simulink model "int2single"  (Simulink 7.6)
settings: Solver=FixedStepDiscrete  StartTime=0.0  StopTime=10000  FixedStep=1  RelTol=1e-3
settings Model: Creator=jordan  LastModifiedBy=jordan
settings DataIOCC: LimitDataPoints=off  SaveOutput=off  SignalLogging=off  DSMLogging=off  SaveTime=off
settings OptimizationCC: BlockReduction=off  ConditionallyExecuteInputs=off

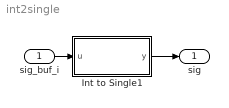
== system int2single ==
  sig_buf_i : Inport  OutDataTypeStr=fixdt(0,12,0)
  Int to Single1 : Stateflow chart  TreatAsAtomicUnit=on
  sig : Outport  OutDataTypeStr=uint32  PortDimensions=1
  wires:
  Int to Single1/1(y) -> sig/1
  sig_buf_i/1 -> Int to Single1/1(u)

== matlab function Int to Single1 ==
  data: u input fixdt(0,12,0); y output uint32
function y = fcn(u)
%#eml

sig=uint8(0);
exp=uint8(0);
frac=fi(0,0,23,0);

%Transform two's complement integer into unnormalized
%single number
buf=fi(0,0,12,0);
sig=uint8(0);
buf=u;
frac1=fi(buf,0,23,0);

%Normalize floating-point number
buf1=fi(frac1,0,24,0);
p=fi(0,0,5,0);
mask=fi(2^22,0,24,0);
for ind=1:23
    c=bitand(buf1,mask);
    if (c==0)
        buf1=bitshift(buf1,1);
        p=fi(p+1,0,5,0);
    end
end
p=fi(p+1,0,5,0);
buf1=bitshift(fi(frac1,0,24,0),uint8(p));
mask1=fi(2^23-1,0,24,0);
buf1=bitand(buf1,mask1);
frac=fi(buf1,0,23,0);
exp=uint8(127+(22-p));

%Compose floating-point number
z=uint32(0);
if sig
    z=uint32(bitshift(uint32(1),31));
end
buf2=uint32(bitshift(uint32(exp),23));
z=bitor(z,buf2);
z=bitor(z,uint32(frac));
y=z;
